simulink model "SimuBFContinuDiscret_regu_PD_2020a"  (R2024b)
settings: Solver=VariableStepAuto  StartTime=0.0  StopTime=10  FixedStep=0.001  RelTol=1e-4
undefined symbols (not defined in the file): A0, den, den_reg, echelon, fs, num_reg, u0, wn, y0, zeta
settings Model: Creator=Admin  LastModifiedBy=ajj
settings SolverCC: AlgebraicLoopSolver=TrustRegion
settings DebuggingCC: UnconnectedInputMsg=warning  UnconnectedOutputMsg=warning  UnconnectedLineMsg=warning
settings ModelReferenceCC: EnableRefExpFcnMdlSchedulingChecks=on
settings RTWCC: GPUComputeCapability=3.5

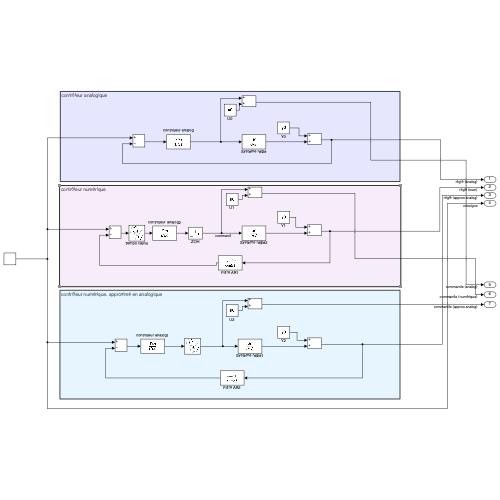
[thumbnail: Simulink's stored preview of the top-level diagram]
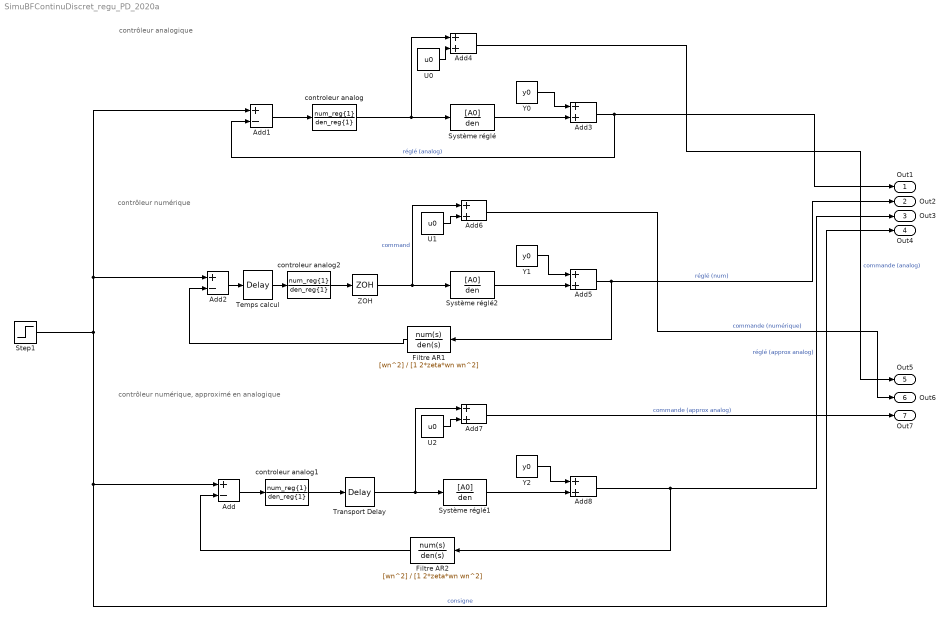
== system SimuBFContinuDiscret_regu_PD_2020a ==
  note: contrôleur numérique, approximé en analogique
  note: contrôleur numérique
  note: contrôleur analogique
  Add : Sum  Inputs=+-
  Add1 : Sum  Inputs=+-
  Add2 : Sum  Inputs=+-
  Add{3..8} (6 alike) : Sum
  Filtre AR1 : TransferFcn  Numerator=[wn^2]  Denominator=[1 2*zeta*wn wn^2]
  Filtre AR2 : TransferFcn  Numerator=[wn^2]  Denominator=[1 2*zeta*wn wn^2]
  Step1 : Step  Before=y0  After=y0+echelon  SampleTime=0
  Système réglé : TransferFcn  Numerator=[A0]  Denominator=den
  Système réglé1 : TransferFcn  Numerator=[A0]  Denominator=den
  Système réglé2 : TransferFcn  Numerator=[A0]  Denominator=den
  Temps calcul : TransportDelay  DelayTime=1/(2*fs)
  Transport Delay : TransportDelay  DelayTime=1/fs
  U0 : Constant  Value=u0
  U1 : Constant  Value=u0
  U2 : Constant  Value=u0
  Y0 : Constant  Value=y0
  Y1 : Constant  Value=y0
  Y2 : Constant  Value=y0
  ZOH : ZeroOrderHold  SampleTime=1/fs
  controleur analog : TransferFcn  Numerator=num_reg{1}  Denominator=den_reg{1}
  controleur analog1 : TransferFcn  Numerator=num_reg{1}  Denominator=den_reg{1}
  controleur analog2 : TransferFcn  Numerator=num_reg{1}  Denominator=den_reg{1}
  Out1 : Outport
  Out2 : Outport  Port=2
  Out3 : Outport  Port=3
  Out4 : Outport  Port=4
  Out5 : Outport  Port=5
  Out6 : Outport  Port=6
  Out7 : Outport  Port=7
  wires:
  Add1/1 -> controleur analog/1
  controleur analog/1 -> Add4/1, Système réglé/1
  ZOH/1 -> Système réglé2/1, Add6/1  "command"
  controleur analog2/1 -> ZOH/1
  Add2/1 -> Temps calcul/1
  Système réglé/1 -> Add3/2
  Filtre AR1/1 -> Add2/2
  controleur analog1/1 -> Transport Delay/1
  Transport Delay/1 -> Système réglé1/1, Add7/1
  Add/1 -> controleur analog1/1
  Filtre AR2/1 -> Add/2
  Step1/1 -> Out4/1, Add/1, Add1/1, Add2/1  "consigne"
  Système réglé1/1 -> Add8/2
  Système réglé2/1 -> Add5/2
  Add3/1 -> Out1/1, Add1/2  "réglé (analog)"
  Y0/1 -> Add3/1
  U0/1 -> Add4/2
  Add4/1 -> Out5/1  "commande (analog)"
  Add5/1 -> Out2/1, Filtre AR1/1  "réglé (num)"
  Y1/1 -> Add5/1
  U1/1 -> Add6/2
  Add6/1 -> Out6/1  "commande (numérique)"
  U2/1 -> Add7/2
  Add7/1 -> Out7/1  "commande (approx analog)"
  Add8/1 -> Out3/1, Filtre AR2/1  "réglé (approx analog)"
  Y2/1 -> Add8/1
  Temps calcul/1 -> controleur analog2/1
